simulink model "ttime_learn1"  (R2017a)
settings: Solver=VariableStepAuto  StartTime=0.0  StopTime=10.0  RelTol=1e-3
undefined symbols (not defined in the file or in its folder): Hz
libraries: truetime x1
settings Model: Creator=erich  LastModifiedBy=erich

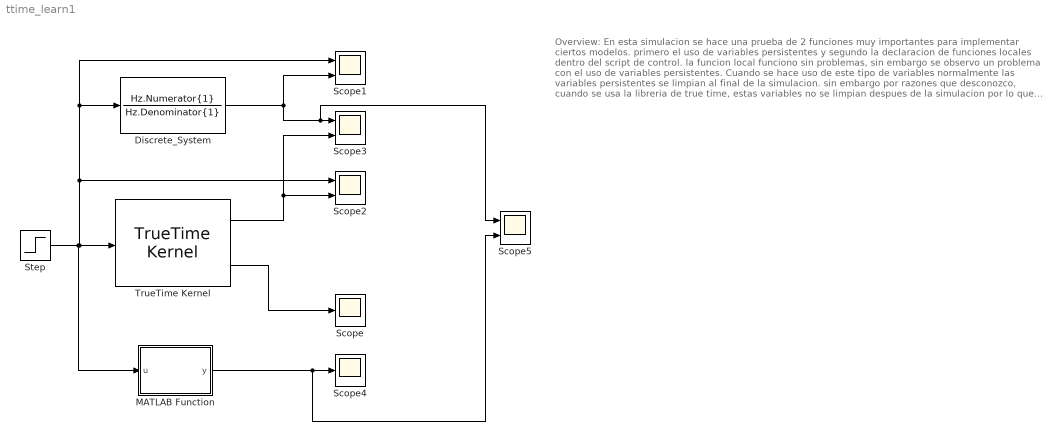
== system ttime_learn1 ==
  note: Overview:
      | En esta simulacion se hace una prueba de 2 funciones muy importantes
      | para implementar ciertos modelos. primero el uso de variables persistentes
      | y segundo la declaracion de funciones locales dentro del script de control.
      |
      | la funcion local funciono sin problemas, sin embargo se observo un
      | problema con el uso de variables persistentes. Cuando se hace uso de
      | este tipo de variables normalmente las variables persistentes se limpian
      | al final de la simulacion. sin embargo por razones que desconozco,
      | cuando se usa la libreria de true time, estas variables no se limpian
      | despues de la simulacion por lo que es necesario limpiarlas manualmente.
      |
      | En este caso la funcion de control es calc.m.
      | para limpiar las variables persistentes es necesario ejecutar el comando
      | >> clear calc.
      |
      | se puede ver que cuando se ejecuta la simulacion 2 veces, la primera
      | simulacion conicide con la funcion de transferencia en z pero la segunda
      | ya no coincide ya que las variables persistentes quedan en memoria.
      | sin embargo, si se ejecuta la segunda vez despues de ejecutar el
      | comando clear calc, la simulacion permance igual.
  Discrete_System : DiscreteTransferFcn  Numerator=Hz.Numerator{1}  Denominator=Hz.Denominator{1}  SampleTime=.1
  MATLAB Function : MATLAB Function  TreatAsAtomicUnit=on  SystemSampleTime=.1
  Scope : Scope
  Scope{1..3,5} (4 alike) : Scope  NumInputPorts=2
  Scope4 : Scope
  Step : Step  SampleTime=0
  TrueTime Kernel : truetime/TrueTime Kernel  sfun=tttest  args=[]  ninputsoutputs=[1 1]  ntriggers=0  trigtype=falling  nwnodenbr=[]  clockoffsetdrift=[0 0]  schedoutput=on  battery=off  poweroutput=off
  wires:
  Step/1 -> MATLAB Function/1(u), Scope2/1, Scope1/1, Discrete_System/1, TrueTime Kernel/1
  TrueTime Kernel/1 -> Scope2/2, Scope3/2
  Discrete_System/1 -> Scope5/1, Scope3/1, Scope1/2
  TrueTime Kernel/2 -> Scope/1
  MATLAB Function/1(y) -> Scope5/2, Scope4/1

== matlab function ttime_learn1/MATLAB Function ==
  data: u input; y output
function y = fcn(u)
persistent U;
if isempty(U)
    U = zeros(1, 3);
end
persistent Y;
if isempty(Y)
    Y = zeros(1, 2);
end
U = [u U(1:end-1)];
y_1 = (3867417694454701*U(2))/36028797018963968 - (6329353517423041*U(3))/72057594037927936 + (4389385923699487*Y(1))/2251799813685248 - (1070989120431317*Y(2))/1125899906842624;
Y = [y_1 Y(1:end-1)];

y = y_1;
